simulink model "wind_turb_AND_pmsm_V2"  (R2016a)
settings: Solver=VariableStepAuto  StartTime=0.0  StopTime=0.25*100e6  RelTol=1e-3
libraries: xbsIndex_r4 x16, powerlib_meascontrol x2
settings Model: Creator=Jorge  LastModifiedBy=Jorge

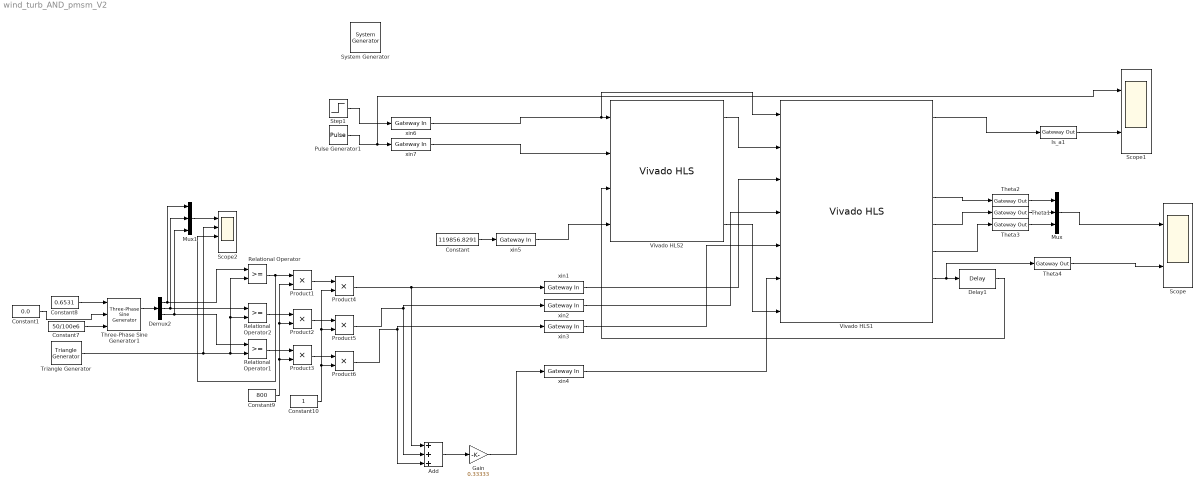
== system wind_turb_AND_pmsm_V2 ==
  " System Generator" : xbsIndex_r4/ System Generator  Tag=genX  xilinxfamily=zynq  part=xc7z020  speed=-1  package=clg400  synthesis_tool=Vivado  clock_wrapper=Clock Enables  directory=./netlist  proj_type=Vivado  Synth_file=Vivado Synthesis Defaults  Impl_file=Vivado Implementation Defaults  testbench=off  simulink_period=1  sysclk_period=10  dcm_input_clock_period=10  incr_netlist=off  trim_vbits=Everywhere in SubSystem  dbl_ovrd=According to Block Masks  core_generation=According to Block Masks  run_coregen=off  deprecated_control=off  eval_field=0  block_type=sysgen
  Add : Sum  Inputs=+++  RndMeth=Nearest
  Constant : Constant  Value=119856.8291
  Constant1 : Constant  Value=0.0
  Constant10 : Constant
  Constant7 : Constant  Value=50/100e6
  Constant8 : Constant  Value=0.6531
  Constant9 : Constant  Value=800
  Delay1 : xbsIndex_r4/Delay  rst=off  infoeditControl=Selection of Reset will increase slice count due to use of real FFs and instead of SRLs  en=off  latency=1  reg_retiming=off  dbl_ovrd=off  block_type=delay
  Demux2 : Demux  Outputs=3
  Gain : Gain  Gain=0.33333
  Is_a1 : xbsIndex_r4/Gateway Out  inherit_from_input=off  hdl_port=on  rows=1  columns=1  UseAsDAC=off  DACChannel='1'  interface=None  automatic_assignment=on  address_offset=hex2dec('00')  intf_name=''  intf_description=''  timing_constraint=None  locs_specified=off  LOCs={}  io_standard={}  block_type=gatewayout
  Mux : Mux  Inputs=3
  Mux1 : Mux  Inputs=3
  Product{1..6} (6 alike) : Product
  Pulse Generator1 : DiscretePulseGenerator  PulseType=Time based  Period=200
  Relational Operator : RelationalOperator  OutDataTypeStr=boolean  ZeroCross=off
  Relational Operator1 : RelationalOperator  OutDataTypeStr=boolean  ZeroCross=off
  Relational Operator2 : RelationalOperator  OutDataTypeStr=boolean  ZeroCross=off
  Scope : Scope  NumInputPorts=2
  Scope1 : Scope  NumInputPorts=2
  Scope2 : Scope  NumInputPorts=4
  Step1 : Step  Time=1e-6  SampleTime=0
  Theta{1..4} (4 alike) : xbsIndex_r4/Gateway Out  inherit_from_input=off  hdl_port=on  rows=1  columns=1  UseAsDAC=off  DACChannel='1'  interface=None  automatic_assignment=on  address_offset=hex2dec('00')  intf_name=''  intf_description=''  timing_constraint=None  locs_specified=off  LOCs={}  io_standard={}  block_type=gatewayout
  Three-Phase Sine Generator1 : powerlib_meascontrol/Pulse & Signal Generators/Three-Phase Sine Generator  Ts=1
  Triangle Generator : powerlib_meascontrol/Pulse & Signal Generators/Triangle Generator  Freq=5e3/100e6  Phase=0  Ts=1
  Vivado HLS1 : xbsIndex_r4/Vivado HLS  anytable='C:/Users/Jorge/Documents/GitHub/nvHIL/hls/pmsm_V2/pmsm_V2_prj/sol_sysgen'  fast_sim=off  display_datatype=on  rate_propagation_method=Simulink system period  model_file_path=''  latency=1  block_type=hls
      settings: infoedit=This block allows including C,C++ and SystemC source files in System Generator for DSP designs.
  Vivado HLS2 : xbsIndex_r4/Vivado HLS  anytable='C:\Users\Jorge\Documents\GitHub\nvHIL\hls\wind_tur_V2\wind_turb_V2_prj\sol_sysgen'  fast_sim=off  display_datatype=on  rate_propagation_method=Simulink system period  model_file_path=''  latency=1  block_type=hls
      settings: infoedit=This block allows including C,C++ and SystemC source files in System Generator for DSP designs.
  xin1 : xbsIndex_r4/Gateway In  gui_display_data_type=Fixed-point  arith_type="Signed  (2's comp)"  n_bits=25  bin_pt=9  preci_type=Single  exp_width=8  frac_width=24  rows=1  columns=1  quantization="Round  (unbiased: +/- Inf)"  overflow=Saturate  period=1  UseAsADC=off  ADCChannel='1'  interface=None  automatic_assignment=on  address_offset=hex2dec('00')  intf_name=''  intf_description=''  default_value=0  timing_constraint=None  locs_specified=off  LOCs={}  io_standard={}  inherit_from_input=off  hdl_port=on  dbl_ovrd=off  block_type=gatewayin
  xin2 : xbsIndex_r4/Gateway In  gui_display_data_type=Fixed-point  arith_type="Signed  (2's comp)"  n_bits=25  bin_pt=9  preci_type=Single  exp_width=8  frac_width=24  rows=1  columns=1  quantization="Round  (unbiased: +/- Inf)"  overflow=Saturate  period=1  UseAsADC=off  ADCChannel='1'  interface=None  automatic_assignment=on  address_offset=hex2dec('00')  intf_name=''  intf_description=''  default_value=0  timing_constraint=None  locs_specified=off  LOCs={}  io_standard={}  inherit_from_input=off  hdl_port=on  dbl_ovrd=off  block_type=gatewayin
  xin3 : xbsIndex_r4/Gateway In  gui_display_data_type=Fixed-point  arith_type="Signed  (2's comp)"  n_bits=25  bin_pt=9  preci_type=Single  exp_width=8  frac_width=24  rows=1  columns=1  quantization="Round  (unbiased: +/- Inf)"  overflow=Saturate  period=1  UseAsADC=off  ADCChannel='1'  interface=None  automatic_assignment=on  address_offset=hex2dec('00')  intf_name=''  intf_description=''  default_value=0  timing_constraint=None  locs_specified=off  LOCs={}  io_standard={}  inherit_from_input=off  hdl_port=on  dbl_ovrd=off  block_type=gatewayin
  xin4 : xbsIndex_r4/Gateway In  gui_display_data_type=Fixed-point  arith_type="Signed  (2's comp)"  n_bits=18  bin_pt=6  preci_type=Single  exp_width=8  frac_width=24  rows=1  columns=1  quantization="Round  (unbiased: +/- Inf)"  overflow=Saturate  period=1  UseAsADC=off  ADCChannel='1'  interface=None  automatic_assignment=on  address_offset=hex2dec('00')  intf_name=''  intf_description=''  default_value=0  timing_constraint=None  locs_specified=off  LOCs={}  io_standard={}  inherit_from_input=off  hdl_port=on  dbl_ovrd=off  block_type=gatewayin
  xin5 : xbsIndex_r4/Gateway In  gui_display_data_type=Fixed-point  arith_type="Signed  (2's comp)"  n_bits=21  bin_pt=1  preci_type=Single  exp_width=8  frac_width=24  rows=1  columns=1  quantization="Round  (unbiased: +/- Inf)"  overflow=Saturate  period=1  UseAsADC=off  ADCChannel='1'  interface=None  automatic_assignment=on  address_offset=hex2dec('00')  intf_name=''  intf_description=''  default_value=0  timing_constraint=None  locs_specified=off  LOCs={}  io_standard={}  inherit_from_input=off  hdl_port=on  dbl_ovrd=off  block_type=gatewayin
  xin6 : xbsIndex_r4/Gateway In  gui_display_data_type=Boolean  arith_type=Boolean  n_bits=16  bin_pt=10  preci_type=Single  exp_width=8  frac_width=24  rows=1  columns=1  quantization="Round  (unbiased: +/- Inf)"  overflow=Saturate  period=1  UseAsADC=off  ADCChannel='1'  interface=None  automatic_assignment=on  address_offset=hex2dec('00')  intf_name=''  intf_description=''  default_value=0  timing_constraint=None  locs_specified=off  LOCs={}  io_standard={}  inherit_from_input=off  hdl_port=on  dbl_ovrd=off  block_type=gatewayin
  xin7 : xbsIndex_r4/Gateway In  gui_display_data_type=Boolean  arith_type=Boolean  n_bits=16  bin_pt=10  preci_type=Single  exp_width=8  frac_width=24  rows=1  columns=1  quantization="Round  (unbiased: +/- Inf)"  overflow=Saturate  period=1  UseAsADC=off  ADCChannel='1'  interface=None  automatic_assignment=on  address_offset=hex2dec('00')  intf_name=''  intf_description=''  default_value=0  timing_constraint=None  locs_specified=off  LOCs={}  io_standard={}  inherit_from_input=off  hdl_port=on  dbl_ovrd=off  block_type=gatewayin
  wires:
  Step1/1 -> xin6/1
  Pulse Generator1/1 -> Scope1/1, xin7/1
  Is_a1/1 -> Scope1/2
  Constant/1 -> xin5/1
  Theta4/1 -> Scope/2
  xin6/1 -> Vivado HLS1/1, Vivado HLS2/1
  xin7/1 -> Vivado HLS2/2
  Vivado HLS2/1 -> Vivado HLS1/2
  Vivado HLS1/1 -> Is_a1/1
  Vivado HLS2/4 -> Vivado HLS1/7
  Delay1/1 -> Vivado HLS2/3
  xin5/1 -> Vivado HLS2/4
  Demux2/1 -> Mux1/1, Relational Operator/1
  Demux2/2 -> Mux1/2, Relational Operator2/1
  Demux2/3 -> Mux1/3, Relational Operator1/1
  Triangle Generator/1 -> Scope2/2, Relational Operator1/2, Relational Operator2/2, Relational Operator/2
  Relational Operator/1 -> Scope2/3, Product1/1
  Relational Operator1/1 -> Product3/1
  Relational Operator2/1 -> Product2/1
  Constant7/1 -> Three-Phase Sine Generator1/3
  Constant8/1 -> Three-Phase Sine Generator1/1
  Three-Phase Sine Generator1/1 -> Demux2/1
  Constant9/1 -> Product3/2, Product2/2, Product1/2
  Product1/1 -> Product4/1
  Product3/1 -> Product6/1
  Product2/1 -> Product5/1
  Constant10/1 -> Product6/2, Product5/2, Product4/2
  Product4/1 -> xin1/1, Add/1
  Product5/1 -> xin2/1, Add/2
  Product6/1 -> xin3/1, Add/3
  Add/1 -> Gain/1
  Mux1/1 -> Scope2/1
  Constant1/1 -> Three-Phase Sine Generator1/2
  xin1/1 -> Vivado HLS1/3
  xin2/1 -> Vivado HLS1/4
  xin3/1 -> Vivado HLS1/5
  xin4/1 -> Vivado HLS1/6
  Gain/1 -> xin4/1
  Vivado HLS1/4 -> Theta2/1
  Vivado HLS1/5 -> Theta1/1
  Vivado HLS1/6 -> Theta3/1
  Mux/1 -> Scope/1
  Theta2/1 -> Mux/1
  Theta1/1 -> Mux/2
  Theta3/1 -> Mux/3
  Vivado HLS1/7 -> Delay1/1, Theta4/1
